simulink model "DynamicsAaa"  (R2017a)
settings: Solver=VariableStepAuto  StartTime=0.0  StopTime=200  RelTol=1e-3
(part 8 of 8)

== matlab function DynamicsAaa/omega ==
  data: q input; wx output; qd input; wy output; wz output
function [wx ,wy, wz] = fcn(q , qd)

q1 = q(1);
q2 = q(2);
q3 = q(3);
q4 = q(4);
q5 = q(5);
q6 = q(6);

c1 = cos(q(1));
c2 = cos(q(2));
c3 = cos(q(3));
c4 = cos(q(4));
c5 = cos(q(5));
c6 = cos(q(6));
s1 = sin(q(1));
s2 = sin(q(2));
s3 = sin(q(3));
s4 = sin(q(4));
s5 = sin(q(5));
s6 = sin(q(6));

wx = c6*(c5*(-c3*s4*(q(1) + q(2)) + c4*s3*(q(1) + q(2))) - s5*(-q(3) + q(4))) - s6*(-c5*(-q(3) + q(4)) - s5*(-c3*s4*(q(1) + q(2)) + c4*s3*(q(1) + q(2))));
  
wy = -c6*(-c5*(-q(3) + q(4)) - s5*(-c3*s4*(q(1) + q(2)) + c4*s3*(q(1) + q(2)))) - s6*(c5*(-c3*s4*(q(1) + q(2)) + c4*s3*(q(1) + q(2))) - s5*(-q(3) + q(4)));
  
wz = c3*c4*(q(1) + q(2)) - q(5) + q(6) + s3*s4*(q(1) + q(2));

== matlab function DynamicsAaa/POSITION ==
  data: q input; px output; py output; pz output
function [px,py,pz] = fcn(q)
%#codegen

q1 = q(1);
q2 = q(2);
q3 = q(3);
q4 = q(4);
q5 = q(5);
q6 = q(6);


px = 270*cos(q(1)) + 90*cos(q(1))*cos(q(2)) - 295*cos(q(1))*sin(q(2)) - 295*cos(q(2))*sin(q(1)) - 90*sin(q(1))*sin(q(2)) + 80*cos(q(3))*sin(q(4))*(cos(q(1))*cos(q(2)) - sin(q(1))*sin(q(2))) - 80*cos(q(4))*sin(q(3))*(cos(q(1))*cos(q(2)) - sin(q(1))*sin(q(2))) + 75;
py = 80*cos(q(3))*cos(q(4)) + 80*sin(q(3))*sin(q(4)) + 335;
pz = 295*sin(q(1))*sin(q(2)) - 295*cos(q(1))*cos(q(2)) - 90*cos(q(1))*sin(q(2)) - 90*cos(q(2))*sin(q(1)) - 270*sin(q(1)) - 80*cos(q(3))*sin(q(4))*(cos(q(1))*sin(q(2)) + cos(q(2))*sin(q(1))) + 80*cos(q(4))*sin(q(3))*(cos(q(1))*sin(q(2)) + cos(q(2))*sin(q(1)));
 

 px;
 py;
 pz

== matlab function DynamicsAaa/Subsystem/Jacobian//Jacobian_dot//X_dot//X_ddot ==
  data: J output; q1 input; J_dot output; qd1 input; q2 input; qd2 input; q3 input; qd3 input; q4 input; qd4 input; q5 input; qd5 input; q6 input; qd6 input; qdd1 input; qdd2 input; qdd3 input; qdd4 input; qdd5 input; qdd6 input; X_dot output; X_ddot output
function [J,J_dot,X_dot,X_ddot] = fcn(q1,qd1,q2,qd2,q3,qd3,q4,qd4,q5,qd5,q6,qd6,qdd1,qdd2,qdd3,qdd4,qdd5,qdd6)
%#codegen

j1 = [ 295*sin(q1)*sin(q2) - 295*cos(q1)*cos(q2) - 90*cos(q1)*sin(q2) - 90*cos(q2)*sin(q1) - 270*sin(q1) - 80*cos(q3)*sin(q4)*(cos(q1)*sin(q2) + cos(q2)*sin(q1)) + 80*cos(q4)*sin(q3)*(cos(q1)*sin(q2) + cos(q2)*sin(q1)), 295*sin(q1)*sin(q2) - 90*cos(q1)*sin(q2) - 90*cos(q2)*sin(q1) - 295*cos(q1)*cos(q2) - 80*cos(q3)*sin(q4)*(cos(q1)*sin(q2) + cos(q2)*sin(q1)) + 80*cos(q4)*sin(q3)*(cos(q1)*sin(q2) + cos(q2)*sin(q1)), - 80*cos(q3)*cos(q4)*(cos(q1)*cos(q2) - sin(q1)*sin(q2)) - 80*sin(q3)*sin(q4)*(cos(q1)*cos(q2) - sin(q1)*sin(q2)),   80*cos(q3)*cos(q4)*(cos(q1)*cos(q2) - sin(q1)*sin(q2)) + 80*sin(q3)*sin(q4)*(cos(q1)*cos(q2) - sin(q1)*sin(q2)), 0, 0];
j2 =[                                                                                                                                                                                                                   0,                                                                                                                                                                                                     0,                                                                           80*cos(q3)*sin(q4) - 80*cos(q4)*sin(q3),                                                                           80*cos(q4)*sin(q3) - 80*cos(q3)*sin(q4), 0, 0];
j3 = [295*cos(q1)*sin(q2) - 90*cos(q1)*cos(q2) - 270*cos(q1) + 295*cos(q2)*sin(q1) + 90*sin(q1)*sin(q2) - 80*cos(q3)*sin(q4)*(cos(q1)*cos(q2) - sin(q1)*sin(q2)) + 80*cos(q4)*sin(q3)*(cos(q1)*cos(q2) - sin(q1)*sin(q2)), 295*cos(q1)*sin(q2) - 90*cos(q1)*cos(q2) + 295*cos(q2)*sin(q1) + 90*sin(q1)*sin(q2) - 80*cos(q3)*sin(q4)*(cos(q1)*cos(q2) - sin(q1)*sin(q2)) + 80*cos(q4)*sin(q3)*(cos(q1)*cos(q2) - sin(q1)*sin(q2)),   80*cos(q3)*cos(q4)*(cos(q1)*sin(q2) + cos(q2)*sin(q1)) + 80*sin(q3)*sin(q4)*(cos(q1)*sin(q2) + cos(q2)*sin(q1)), - 80*cos(q3)*cos(q4)*(cos(q1)*sin(q2) + cos(q2)*sin(q1)) - 80*sin(q3)*sin(q4)*(cos(q1)*sin(q2) + cos(q2)*sin(q1)), 0, 0];
 
J = [j1;j2;j3];

j1_dot = [ qd1*(295*cos(q1)*sin(q2) - 90*cos(q1)*cos(q2) - 270*cos(q1) + 295*cos(q2)*sin(q1) + 90*sin(q1)*sin(q2) - 80*cos(q3)*sin(q4)*(cos(q1)*cos(q2) - sin(q1)*sin(q2)) + 80*cos(q4)*sin(q3)*(cos(q1)*cos(q2) - sin(q1)*sin(q2))) + qd3*(80*cos(q3)*cos(q4)*(cos(q1)*sin(q2) + cos(q2)*sin(q1)) + 80*sin(q3)*sin(q4)*(cos(q1)*sin(q2) + cos(q2)*sin(q1))) - qd4*(80*cos(q3)*cos(q4)*(cos(q1)*sin(q2) + cos(q2)*sin(q1)) + 80*sin(q3)*sin(q4)*(cos(q1)*sin(q2) + cos(q2)*sin(q1))) + qd2*(295*cos(q1)*sin(q2) - 90*cos(q1)*cos(q2) + 295*cos(q2)*sin(q1) + 90*sin(q1)*sin(q2) - 80*cos(q3)*sin(q4)*(cos(q1)*cos(q2) - sin(q1)*sin(q2)) + 80*cos(q4)*sin(q3)*(cos(q1)*cos(q2) - sin(q1)*sin(q2))), qd3*(80*cos(q3)*cos(q4)*(cos(q1)*sin(q2) + cos(q2)*sin(q1)) + 80*sin(q3)*sin(q4)*(cos(q1)*sin(q2) + cos(q2)*sin(q1))) - qd4*(80*cos(q3)*cos(q4)*(cos(q1)*sin(q2) + cos(q2)*sin(q1)) + 80*sin(q3)*sin(q4)*(cos(q1)*sin(q2) + cos(q2)*sin(q1))) + qd1*(295*cos(q1)*sin(q2) - 90*cos(q1)*cos(q2) + 295*cos(q2)*sin(q1) + 90*sin(q1)*sin(q2) - 80*cos(q3)*sin(q4)*(cos(q1)*cos(q2) - sin(q1)*sin(q2)) + 80*cos(q4)*sin(q3)*(cos(q1)*cos(q2) - sin(q1)*sin(q2))) + qd2*(295*cos(q1)*sin(q2) - 90*cos(q1)*cos(q2) + 295*cos(q2)*sin(q1) + 90*sin(q1)*sin(q2) - 80*cos(q3)*sin(q4)*(cos(q1)*cos(q2) - sin(q1)*sin(q2)) + 80*cos(q4)*sin(q3)*(cos(q1)*cos(q2) - sin(q1)*sin(q2))), qd1*(80*cos(q3)*cos(q4)*(cos(q1)*sin(q2) + cos(q2)*sin(q1)) + 80*sin(q3)*sin(q4)*(cos(q1)*sin(q2) + cos(q2)*sin(q1))) + qd2*(80*cos(q3)*cos(q4)*(cos(q1)*sin(q2) + cos(q2)*sin(q1)) + 80*sin(q3)*sin(q4)*(cos(q1)*sin(q2) + cos(q2)*sin(q1))) - qd3*(80*cos(q3)*sin(q4)*(cos(q1)*cos(q2) - sin(q1)*sin(q2)) - 80*cos(q4)*sin(q3)*(cos(q1)*cos(q2) - sin(q1)*sin(q2))) + qd4*(80*cos(q3)*sin(q4)*(cos(q1)*cos(q2) - sin(q1)*sin(q2)) - 80*cos(q4)*sin(q3)*(cos(q1)*cos(q2) - sin(q1)*sin(q2))), qd3*(80*cos(q3)*sin(q4)*(cos(q1)*cos(q2) - sin(q1)*sin(q2)) - 80*cos(q4)*sin(q3)*(cos(q1)*cos(q2) - sin(q1)*sin(q2))) - qd2*(80*cos(q3)*cos(q4)*(cos(q1)*sin(q2) + cos(q2)*sin(q1)) + 80*sin(q3)*sin(q4)*(cos(q1)*sin(q2) + cos(q2)*sin(q1))) - qd1*(80*cos(q3)*cos(q4)*(cos(q1)*sin(q2) + cos(q2)*sin(q1)) + 80*sin(q3)*sin(q4)*(cos(q1)*sin(q2) + cos(q2)*sin(q1))) - qd4*(80*cos(q3)*sin(q4)*(cos(q1)*cos(q2) - sin(q1)*sin(q2)) - 80*cos(q4)*sin(q3)*(cos(q1)*cos(q2) - sin(q1)*sin(q2))), 0, 0];
j2_dot = [                                                                                                                                                                                                                                                                                                                                                                                                                                                                                                                                                                                                                                                                                                   0,                                                                                                                                                                                                                                                                                                                                                                                                                                                                                                                                                                                                                                                                                     0,                                                                                                                                                                                                                                                                                                                                                                                                       qd4*(80*cos(q3)*cos(q4) + 80*sin(q3)*sin(q4)) - qd3*(80*cos(q3)*cos(q4) + 80*sin(q3)*sin(q4)),                                                                                                                                                                                                                                                                                                                                                                                                       qd3*(80*cos(q3)*cos(q4) + 80*sin(q3)*sin(q4)) - qd4*(80*cos(q3)*cos(q4) + 80*sin(q3)*sin(q4)), 0, 0];
j3_dot = [ qd1*(270*sin(q1) + 295*cos(q1)*cos(q2) + 90*cos(q1)*sin(q2) + 90*cos(q2)*sin(q1) - 295*sin(q1)*sin(q2) + 80*cos(q3)*sin(q4)*(cos(q1)*sin(q2) + cos(q2)*sin(q1)) - 80*cos(q4)*sin(q3)*(cos(q1)*sin(q2) + cos(q2)*sin(q1))) + qd3*(80*cos(q3)*cos(q4)*(cos(q1)*cos(q2) - sin(q1)*sin(q2)) + 80*sin(q3)*sin(q4)*(cos(q1)*cos(q2) - sin(q1)*sin(q2))) - qd4*(80*cos(q3)*cos(q4)*(cos(q1)*cos(q2) - sin(q1)*sin(q2)) + 80*sin(q3)*sin(q4)*(cos(q1)*cos(q2) - sin(q1)*sin(q2))) + qd2*(295*cos(q1)*cos(q2) + 90*cos(q1)*sin(q2) + 90*cos(q2)*sin(q1) - 295*sin(q1)*sin(q2) + 80*cos(q3)*sin(q4)*(cos(q1)*sin(q2) + cos(q2)*sin(q1)) - 80*cos(q4)*sin(q3)*(cos(q1)*sin(q2) + cos(q2)*sin(q1))), qd3*(80*cos(q3)*cos(q4)*(cos(q1)*cos(q2) - sin(q1)*sin(q2)) + 80*sin(q3)*sin(q4)*(cos(q1)*cos(q2) - sin(q1)*sin(q2))) - qd4*(80*cos(q3)*cos(q4)*(cos(q1)*cos(q2) - sin(q1)*sin(q2)) + 80*sin(q3)*sin(q4)*(cos(q1)*cos(q2) - sin(q1)*sin(q2))) + qd1*(295*cos(q1)*cos(q2) + 90*cos(q1)*sin(q2) + 90*cos(q2)*sin(q1) - 295*sin(q1)*sin(q2) + 80*cos(q3)*sin(q4)*(cos(q1)*sin(q2) + cos(q2)*sin(q1)) - 80*cos(q4)*sin(q3)*(cos(q1)*sin(q2) + cos(q2)*sin(q1))) + qd2*(295*cos(q1)*cos(q2) + 90*cos(q1)*sin(q2) + 90*cos(q2)*sin(q1) - 295*sin(q1)*sin(q2) + 80*cos(q3)*sin(q4)*(cos(q1)*sin(q2) + cos(q2)*sin(q1)) - 80*cos(q4)*sin(q3)*(cos(q1)*sin(q2) + cos(q2)*sin(q1))), qd1*(80*cos(q3)*cos(q4)*(cos(q1)*cos(q2) - sin(q1)*sin(q2)) + 80*sin(q3)*sin(q4)*(cos(q1)*cos(q2) - sin(q1)*sin(q2))) + qd3*(80*cos(q3)*sin(q4)*(cos(q1)*sin(q2) + cos(q2)*sin(q1)) - 80*cos(q4)*sin(q3)*(cos(q1)*sin(q2) + cos(q2)*sin(q1))) + qd2*(80*cos(q3)*cos(q4)*(cos(q1)*cos(q2) - sin(q1)*sin(q2)) + 80*sin(q3)*sin(q4)*(cos(q1)*cos(q2) - sin(q1)*sin(q2))) - qd4*(80*cos(q3)*sin(q4)*(cos(q1)*sin(q2) + cos(q2)*sin(q1)) - 80*cos(q4)*sin(q3)*(cos(q1)*sin(q2) + cos(q2)*sin(q1))), qd4*(80*cos(q3)*sin(q4)*(cos(q1)*sin(q2) + cos(q2)*sin(q1)) - 80*cos(q4)*sin(q3)*(cos(q1)*sin(q2) + cos(q2)*sin(q1))) - qd3*(80*cos(q3)*sin(q4)*(cos(q1)*sin(q2) + cos(q2)*sin(q1)) - 80*cos(q4)*sin(q3)*(cos(q1)*sin(q2) + cos(q2)*sin(q1))) - qd2*(80*cos(q3)*cos(q4)*(cos(q1)*cos(q2) - sin(q1)*sin(q2)) + 80*sin(q3)*sin(q4)*(cos(q1)*cos(q2) - sin(q1)*sin(q2))) - qd1*(80*cos(q3)*cos(q4)*(cos(q1)*cos(q2) - sin(q1)*sin(q2)) + 80*sin(q3)*sin(q4)*(cos(q1)*cos(q2) - sin(q1)*sin(q2))), 0, 0];

J_dot = [j1_dot;j2_dot;j3_dot];


X_dot = J*[qd1 ; qd2 ; qd3 ; qd4 ; qd5 ; qd6 ];
X_ddot = J_dot*[qd1 ; qd2 ; qd3 ; qd4 ; qd5 ; qd6] + J*[qdd1 ; qdd2 ; qdd3 ; qdd4 ; qdd5 ; qdd6];

== matlab function DynamicsAaa/Subsystem/MATLAB Function4 ==
  data: q input; q1 output; qd input; qd1 output; q2 output; qd2 output; q3 output; qd3 output; qdd input; q4 output; qd4 output; q5 output; qd5 output; q6 output; qd6 output; qdd1 output; qdd2 output; qdd3 output; qdd4 output; qdd5 output; qdd6 output
function [q1,qd1,q2,qd2,q3,qd3,q4,qd4,q5,qd5,q6,qd6,qdd1,qdd2,qdd3,qdd4,qdd5,qdd6] = fcn(q,qd,qdd)
%#codegen

q1 = q(1);
q2 = q(2);
q3 = q(3);
q4 = q(4);
q5 = q(5);
q6 = q(6);

qd1 = qd(1);
qd2 = qd(2);
qd3 = qd(3);
qd4 = qd(4);
qd5 = qd(5);
qd6 = qd(6);

qdd1 = qdd(1);
qdd2 = qdd(2);
qdd3 = qdd(3);
qdd4 = qdd(4);
qdd5 = qdd(5);
qdd6 = qdd(6);

== matlab function DynamicsAaa/omegadot ==
  data: q input; wdotx output; qd input; wdoty output; wdotz output; qdd input
function [wdotx ,wdoty, wdotz] = fcn(q , qd, qdd)

q1 = q(1);
q2 = q(2);
q3 = q(3);
q4 = q(4);
q5 = q(5);
q6 = q(6);

c1 = cos(q(1));
c2 = cos(q(2));
c3 = cos(q(3));
c4 = cos(q(4));
c5 = cos(q(5));
c6 = cos(q(6));
s1 = sin(q(1));
s2 = sin(q(2));
s3 = sin(q(3));
s4 = sin(q(4));
s5 = sin(q(5));
s6 = sin(q(6));

wdotx = c6*(c5*(c4*(c3*qd(3)*(qd(1) + qd(2)) + s3*(qdd(1) + qdd(2))) + qd(4)*(-c3*c4*(qd(1) + qd(2)) - s3*s4*(qd(1) + qd(2))) - s4*(c3*(qdd(1) + qdd(2)) - qd(3)*s3*(qd(1) + qd(2)))) + qd(5)*(-c5*(-qd(3) + qd(4)) - s5*(-c3*s4*(qd(1) + qd(2)) + c4*s3*(qd(1) + qd(2)))) - s5*(-qdd(3) + qdd(4))) + qd(6)*(-c6*(-c5*(-qd(3) + qd(4)) - s5*(-c3*s4*(qd(1) + qd(2)) + c4*s3*(qd(1) + qd(2)))) - s6*(c5*(-c3*s4*(qd(1) + qd(2)) + c4*s3*(qd(1) + qd(2))) - s5*(-qd(3) + qd(4)))) - s6*(-c5*(-qdd(3) + qdd(4)) - qd(5)*(c5*(-c3*s4*(qd(1) + qd(2)) + c4*s3*(qd(1) + qd(2))) - s5*(-qd(3) + qd(4))) - s5*(c4*(c3*qd(3)*(qd(1) + qd(2)) + s3*(qdd(1) + qdd(2))) + qd(4)*(-c3*c4*(qd(1) + qd(2)) - s3*s4*(qd(1) + qd(2))) - s4*(c3*(qdd(1) + qdd(2)) - qd(3)*s3*(qd(1) + qd(2)))));
wdoty = -c6*(-c5*(-qdd(3) + qdd(4)) - qd(5)*(c5*(-c3*s4*(qd(1) + qd(2)) + c4*s3*(qd(1) + qd(2))) - s5*(-qd(3) + qd(4))) - s5*(c4*(c3*qd(3)*(qd(1) + qd(2)) + s3*(qdd(1) + qdd(2))) + qd(4)*(-c3*c4*(qd(1) + qd(2)) - s3*s4*(qd(1) + qd(2))) - s4*(c3*(qdd(1) + qdd(2)) - qd(3)*s3*(qd(1) + qd(2))))) - qd(6)*(c6*(c5*(-c3*s4*(qd(1) + qd(2)) + c4*s3*(qd(1) + qd(2))) - s5*(-qd(3) + qd(4))) - s6*(-c5*(-qd(3) + qd(4)) - s5*(-c3*s4*(qd(1) + qd(2)) + c4*s3*(qd(1) + qd(2))))) - s6*(c5*(c4*(c3*qd(3)*(qd(1) + qd(2)) + s3*(qdd(1) + qdd(2))) + qd(4)*(-c3*c4*(qd(1) + qd(2)) - s3*s4*(qd(1) + qd(2))) - s4*(c3*(qdd(1) + qdd(2)) - qd(3)*s3*(qd(1) + qd(2)))) + qd(5)*(-c5*(-qd(3) + qd(4)) - s5*(-c3*s4*(qd(1) + qd(2)) + c4*s3*(qd(1) + qd(2)))) - s5*(-qdd(3) + qdd(4)));
  
wdotz = c4*(c3*(qdd(1) + qdd(2)) - qd(3)*s3*(qd(1) + qd(2))) + qd(4)*(-c3*s4*(qd(1) + qd(2)) + c4*s3*(qd(1) + qd(2))) - qdd(5) + qdd(6) + s4*(c3*qd(3)*(qd(1) + qd(2)) + s3*(qdd(1) + qdd(2)));
